simulink model "version4_dq"  (R2023b)
settings: Solver=VariableStepAuto  StartTime=0.0  StopTime=40  FixedStep=Ts_power  MaxStep=Ts_power  RelTol=1e-3
undefined symbols (not defined in the file): C_dc, c_dc, c_drt, c_f, C_hv_km, C_p_opt, Cagg, Cbase1v, H_gen, H_vsm, H_WTR, Ibase_hv, Ibase_lv, Ibase_mv, k_d_vsm, k_drt, k_p_p_vsm, k_p_q_vsm, K_pitch, ki_q, Kp_cc, kp_dc, kpu, L_comp, L_d, l_f, l_grid, L_hv_km, L_q, l_t_ehvhv, l_t_hvmv, l_t_mvlv, Lagg, lambda_opt, Lbase1v, length_export, omega_nom, omega_WTR_min, omega_WTR_n, omega_WTR_sl, phase_shift_test_state, phase_shifts, pie_export, pitch_max, pitch_min, Pitchanglevector, Powercoefficient, psi_pm, R_a, r_f, r_grid, R_hv_km, r_t_ehvhv, r_t_hvmv, r_t_mvlv, R_WTR, Ragg, rate_max, rate_min, rocof_slope ... (+22)
libraries: slpidlib x6, simulink x2, spsFirstOrderFilterLib x1, spsSampleandHoldLib x1
(part 2 of 3)

== system version4_dq/GFM+WT/CurrentControl ==
  ref : Inport
  meas : Inport  Port=2
  V grid meas : Inport  Port=3
  Constant : Constant
  Demux : Demux  Outputs=2
  Demux1 : Demux  Outputs=2
  Demux2 : Demux  Outputs=3
  Divide1 : Product  Inputs=**
  Divide2 : Product  Inputs=**
  Gain4 : Gain  Gain=l_f
  Gain5 : Gain  Gain=l_f
  Mux : Mux  Inputs=2
  Mux1 : Mux  Inputs=3
  Mux2 : Mux  Inputs=3
  PID Controller : slpidlib/PID Controller  Controller=PI  Form=Ideal  TimeDomain=Continuous-time  UseExternalTs=off  SampleTime=-1  IntegratorMethod=Forward Euler  FilterMethod=Forward Euler  ControllerParametersSource=internal  P=Kp_cc  I=1/Ti_cc  UseKiTs=off  D=0  N=100  UseFilter=on  TunerSelectOption=Transfer Function Based (PID Tuner App)  InitialConditionSource=internal  InitialConditionForIntegrator=0  InitialConditionForFilter=0  DifferentiatorICPrevScaledInput=0  ExternalReset=none  TrackingMode=off  Kt=1  LimitOutput=off  SatLimitsSource=internal  UpperSaturationLimit=inf  LowerSaturationLimit=-inf  LinearizeAsGain=on  AntiWindupMode=none  Kb=1  LimitIntegrator=off  UpperIntegratorSaturationLimit=inf  LowerIntegratorSaturationLimit=-inf  POutMin=[]  POutMax=[]  IOutMin=[]  IOutMax=[]  DOutMin=[]  DOutMax=[]  NOutMin=[]  NOutMax=[]  SumOutMin=[]  SumOutMax=[]  SaturationOutMin=[]  SaturationOutMax=[]  PParamMin=[]  PParamMax=[]  IParamMin=[]  IParamMax=[]  DParamMin=[]  DParamMax=[]  NParamMin=[]  NParamMax=[]  KbParamMin=[]  KbParamMax=[]  KtParamMin=[]  KtParamMax=[]  KbOutMin=[]  KbOutMax=[]  KtOutMin=[]  KtOutMax=[]  IntegratorOutMin=[]  IntegratorOutMax=[]  FilterOutMin=[]  FilterOutMax=[]  SumI1OutMin=[]  SumI1OutMax=[]  SumI2OutMin=[]  SumI2OutMax=[]  SumI3OutMin=[]  SumI3OutMax=[]  SumI4OutMin=[]  SumI4OutMax=[]  SumDOutMin=[]  SumDOutMax=[]  DifferentiatorOutMin=[]  DifferentiatorOutMax=[]  FilterDiffOutCoefMin=[]  FilterDiffOutCoefMax=[]  ReciprocalOutMin=[]  ReciprocalOutMax=[]  SumDenOutMin=[]  SumDenOutMax=[]  SumNumOutMin=[]  SumNumOutMax=[]  DivideOutMin=[]  DivideOutMax=[]  UdiffTsProdOutMin=[]  UdiffTsProdOutMax=[]  NTsProdOutMin=[]  NTsProdOutMax=[]  UintegralTsProdOutMin=[]  UintegralTsProdOutMax=[]  UngainTsProdOutMin=[]  UngainTsProdOutMax=[]  ClampingZeroOutDataTypeStr=Inherit: Inherit via back propagation  ClampingZeroOutMin=[]  ClampingZeroOutMax=[]  FilterDenConstantOutDataTypeStr=Inherit: Inherit via back propagation  FilterDenConstantOutMin=[]  FilterDenConstantOutMax=[]  PCopyOutDataTypeStr=Inherit: Inherit via back propagation  PCopyOutMin=[]  PCopyOutMax=[]  NCopyOutDataTypeStr=Inherit: Inherit via back propagation  NCopyOutMin=[]  NCopyOutMax=[]  IntegratorContinuousStateAttributes='Delta_v_t_q'  IntegratorStateMustResolveToSignalObject=off  IntegratorRTWStateStorageClass=Auto  FilterContinuousStateAttributes=''  FilterStateMustResolveToSignalObject=off  FilterRTWStateStorageClass=Auto  ParallelPVariant=Passthrough  IdealPVariant=InternalParameters  IVariant=InternalParameters  DVariant=Disabled  IntegratorVariant=Continuous  SatVariant=Disabled  AWVariant=Passthrough  PCopyVariant=Disabled  TRVariant=Disabled  FdbkBlocksVariant=Forward  IdealPFdbkVariant=Disabled  SatFdbkVariant=Disabled  DerivativeFilterVariant=Disabled  NVariant=Disabled  NCopyVariant=Disabled_SignalSpec  FilterICVariant=Disabled  IntegratorICVariant=InternalICs  ExternalResetVariant=Disabled  TRSumVariant=Passthrough  SumFdbkVariant=Disabled  SumVariant=Sum_PI  TsampFilterVariant=InternalTs  TsampNgainVariant=Passthrough  TsampIntegralVariant=Disabled_SignalSpec  ExternalSaturationOutDataTypeStr=Inherit: Same as second input
  PID Controller1 : slpidlib/PID Controller  Controller=PI  Form=Ideal  TimeDomain=Continuous-time  UseExternalTs=off  SampleTime=-1  IntegratorMethod=Forward Euler  FilterMethod=Forward Euler  ControllerParametersSource=internal  P=Kp_cc  I=1/Ti_cc  UseKiTs=off  D=0  N=100  UseFilter=on  TunerSelectOption=Transfer Function Based (PID Tuner App)  InitialConditionSource=internal  InitialConditionForIntegrator=1  InitialConditionForFilter=0  DifferentiatorICPrevScaledInput=0  ExternalReset=none  TrackingMode=off  Kt=1  LimitOutput=off  SatLimitsSource=internal  UpperSaturationLimit=inf  LowerSaturationLimit=-inf  LinearizeAsGain=on  AntiWindupMode=none  Kb=1  LimitIntegrator=off  UpperIntegratorSaturationLimit=inf  LowerIntegratorSaturationLimit=-inf  POutMin=[]  POutMax=[]  IOutMin=[]  IOutMax=[]  DOutMin=[]  DOutMax=[]  NOutMin=[]  NOutMax=[]  SumOutMin=[]  SumOutMax=[]  SaturationOutMin=[]  SaturationOutMax=[]  PParamMin=[]  PParamMax=[]  IParamMin=[]  IParamMax=[]  DParamMin=[]  DParamMax=[]  NParamMin=[]  NParamMax=[]  KbParamMin=[]  KbParamMax=[]  KtParamMin=[]  KtParamMax=[]  KbOutMin=[]  KbOutMax=[]  KtOutMin=[]  KtOutMax=[]  IntegratorOutMin=[]  IntegratorOutMax=[]  FilterOutMin=[]  FilterOutMax=[]  SumI1OutMin=[]  SumI1OutMax=[]  SumI2OutMin=[]  SumI2OutMax=[]  SumI3OutMin=[]  SumI3OutMax=[]  SumI4OutMin=[]  SumI4OutMax=[]  SumDOutMin=[]  SumDOutMax=[]  DifferentiatorOutMin=[]  DifferentiatorOutMax=[]  FilterDiffOutCoefMin=[]  FilterDiffOutCoefMax=[]  ReciprocalOutMin=[]  ReciprocalOutMax=[]  SumDenOutMin=[]  SumDenOutMax=[]  SumNumOutMin=[]  SumNumOutMax=[]  DivideOutMin=[]  DivideOutMax=[]  UdiffTsProdOutMin=[]  UdiffTsProdOutMax=[]  NTsProdOutMin=[]  NTsProdOutMax=[]  UintegralTsProdOutMin=[]  UintegralTsProdOutMax=[]  UngainTsProdOutMin=[]  UngainTsProdOutMax=[]  ClampingZeroOutDataTypeStr=Inherit: Inherit via back propagation  ClampingZeroOutMin=[]  ClampingZeroOutMax=[]  FilterDenConstantOutDataTypeStr=Inherit: Inherit via back propagation  FilterDenConstantOutMin=[]  FilterDenConstantOutMax=[]  PCopyOutDataTypeStr=Inherit: Inherit via back propagation  PCopyOutMin=[]  PCopyOutMax=[]  NCopyOutDataTypeStr=Inherit: Inherit via back propagation  NCopyOutMin=[]  NCopyOutMax=[]  IntegratorContinuousStateAttributes='Delta_v_t_d'  IntegratorStateMustResolveToSignalObject=off  IntegratorRTWStateStorageClass=Auto  FilterContinuousStateAttributes=''  FilterStateMustResolveToSignalObject=off  FilterRTWStateStorageClass=Auto  ParallelPVariant=Passthrough  IdealPVariant=InternalParameters  IVariant=InternalParameters  DVariant=Disabled  IntegratorVariant=Continuous  SatVariant=Disabled  AWVariant=Passthrough  PCopyVariant=Disabled  TRVariant=Disabled  FdbkBlocksVariant=Forward  IdealPFdbkVariant=Disabled  SatFdbkVariant=Disabled  DerivativeFilterVariant=Disabled  NVariant=Disabled  NCopyVariant=Disabled_SignalSpec  FilterICVariant=Disabled  IntegratorICVariant=InternalICs  ExternalResetVariant=Disabled  TRSumVariant=Passthrough  SumFdbkVariant=Disabled  SumVariant=Sum_PI  TsampFilterVariant=InternalTs  TsampNgainVariant=Passthrough  TsampIntegralVariant=Disabled_SignalSpec  ExternalSaturationOutDataTypeStr=Inherit: Same as second input
  Step1 : Step  Before=1  SampleTime=0
  Step2 : Step  Before=1  SampleTime=0
  Sum1 : Sum  Inputs=|+-
  Sum2 : Sum  Inputs=+-|
  Sum4 : Sum  Inputs=++-
  Sum5 : Sum  Inputs=+++
  Transfer Fcn2 : TransferFcn  Commented=on  Denominator=[0.005 1]
  Transfer Fcn3 : TransferFcn  Commented=on  Denominator=[0.005 1]
  d-axis-control : Scope  Commented=on  NumInputPorts=3
  q-axis control : Scope  Commented=on  NumInputPorts=3
  v_m : Outport
  wires:
  Mux/1 -> v_m/1
  Sum1/1 -> Divide2/1, d-axis-control/1
  ref/1 -> Demux/1
  meas/1 -> Demux1/1
  Demux1/2 -> Gain5/1, Sum2/2
  Demux1/1 -> Gain4/1, Sum1/2
  Demux/2 -> Sum2/1
  Demux/1 -> Sum1/1
  PID Controller/1 -> Mux2/2, Sum5/2
  Sum4/1 -> d-axis-control/3, Mux/1
  Gain5/1 -> Mux1/3, Sum4/3
  Gain4/1 -> Mux2/3, Sum5/1
  Demux2/2 -> Transfer Fcn3/1
  Sum5/1 -> q-axis control/3, Mux/2
  V grid meas/1 -> Demux2/1
  Demux2/1 -> Transfer Fcn2/1
  Transfer Fcn2/1 -> Mux1/1, Sum4/1
  Mux1/1 -> d-axis-control/2
  Mux2/1 -> q-axis control/2
  Transfer Fcn3/1 -> Mux2/1, Sum5/3
  PID Controller1/1 -> Sum4/2, Mux1/2
  Sum2/1 -> q-axis control/1, Divide1/1
  Step2/1 -> Divide1/2
  Divide1/1 -> PID Controller/1
  Step1/1 -> Divide2/2
  Divide2/1 -> PID Controller1/1

== system version4_dq/GFM+WT/DC-link voltage controller ==
  ref : Inport
  meas : Inport  Port=2
  Mux : Mux  Inputs=2
  PID Controller : slpidlib/PID Controller  Controller=PI  Form=Ideal  TimeDomain=Continuous-time  UseExternalTs=off  SampleTime=-1  IntegratorMethod=Forward Euler  FilterMethod=Forward Euler  ControllerParametersSource=internal  P=kp_dc  I=1/Ti_dc  UseKiTs=off  D=0.0506  N=100  UseFilter=on  TunerSelectOption=Transfer Function Based (PID Tuner App)  InitialConditionSource=internal  InitialConditionForIntegrator=0  InitialConditionForFilter=0  DifferentiatorICPrevScaledInput=0  ExternalReset=none  TrackingMode=off  Kt=1  LimitOutput=off  SatLimitsSource=internal  UpperSaturationLimit=0.5  LowerSaturationLimit=-0.5  LinearizeAsGain=on  AntiWindupMode=clamping  Kb=1  LimitIntegrator=off  UpperIntegratorSaturationLimit=0.5  LowerIntegratorSaturationLimit=-0.5  POutMin=[]  POutMax=[]  IOutMin=[]  IOutMax=[]  DOutMin=[]  DOutMax=[]  NOutMin=[]  NOutMax=[]  SumOutMin=[]  SumOutMax=[]  SaturationOutMin=[]  SaturationOutMax=[]  PParamMin=[]  PParamMax=[]  IParamMin=[]  IParamMax=[]  DParamMin=[]  DParamMax=[]  NParamMin=[]  NParamMax=[]  KbParamMin=[]  KbParamMax=[]  KtParamMin=[]  KtParamMax=[]  KbOutMin=[]  KbOutMax=[]  KtOutMin=[]  KtOutMax=[]  IntegratorOutMin=[]  IntegratorOutMax=[]  FilterOutMin=[]  FilterOutMax=[]  SumI1OutMin=[]  SumI1OutMax=[]  SumI2OutMin=[]  SumI2OutMax=[]  SumI3OutMin=[]  SumI3OutMax=[]  SumI4OutMin=[]  SumI4OutMax=[]  SumDOutMin=[]  SumDOutMax=[]  DifferentiatorOutMin=[]  DifferentiatorOutMax=[]  FilterDiffOutCoefMin=[]  FilterDiffOutCoefMax=[]  ReciprocalOutMin=[]  ReciprocalOutMax=[]  SumDenOutMin=[]  SumDenOutMax=[]  SumNumOutMin=[]  SumNumOutMax=[]  DivideOutMin=[]  DivideOutMax=[]  UdiffTsProdOutMin=[]  UdiffTsProdOutMax=[]  NTsProdOutMin=[]  NTsProdOutMax=[]  UintegralTsProdOutMin=[]  UintegralTsProdOutMax=[]  UngainTsProdOutMin=[]  UngainTsProdOutMax=[]  ClampingZeroOutDataTypeStr=Inherit: Inherit via back propagation  ClampingZeroOutMin=[]  ClampingZeroOutMax=[]  FilterDenConstantOutDataTypeStr=Inherit: Inherit via back propagation  FilterDenConstantOutMin=[]  FilterDenConstantOutMax=[]  PCopyOutDataTypeStr=Inherit: Inherit via back propagation  PCopyOutMin=[]  PCopyOutMax=[]  NCopyOutDataTypeStr=Inherit: Inherit via back propagation  NCopyOutMin=[]  NCopyOutMax=[]  IntegratorContinuousStateAttributes='Delta_P_msc'  IntegratorStateMustResolveToSignalObject=off  IntegratorRTWStateStorageClass=Auto  FilterContinuousStateAttributes=''  FilterStateMustResolveToSignalObject=off  FilterRTWStateStorageClass=Auto  ParallelPVariant=Passthrough  IdealPVariant=InternalParameters  IVariant=InternalParameters  DVariant=Disabled  IntegratorVariant=Continuous  SatVariant=Disabled  AWVariant=Passthrough  PCopyVariant=Disabled  TRVariant=Disabled  FdbkBlocksVariant=Forward  IdealPFdbkVariant=Disabled  SatFdbkVariant=Disabled  DerivativeFilterVariant=Disabled  NVariant=Disabled  NCopyVariant=Disabled_SignalSpec  FilterICVariant=Disabled  IntegratorICVariant=InternalICs  ExternalResetVariant=Disabled  TRSumVariant=Passthrough  SumFdbkVariant=Disabled  SumVariant=Sum_PI  TsampFilterVariant=InternalTs  TsampNgainVariant=Passthrough  TsampIntegralVariant=Disabled_SignalSpec  ExternalSaturationOutDataTypeStr=Inherit: Same as second input
  Square : Math  Operator=square
  Square1 : Math  Operator=square
  Sum : Sum  Inputs=+-|
  input : Outport
  error : Outport  Port=2
  out : Outport  Port=3
  Out4 : Outport  Port=4
  wires:
  Mux/1 -> input/1
  PID Controller/1 -> Out4/1, out/1
  meas/1 -> Square/1
  ref/1 -> Square1/1
  Square/1 -> Mux/2, Sum/2
  Square1/1 -> Mux/1, Sum/1
  Sum/1 -> PID Controller/1, error/1

== system version4_dq/GFM+WT/PLL>>grid1 ==
  note: inv ([  cos(wt)   sin(wt)
      |    -sin(wt)    cos(wt)   ])
  note: =
  note: [  al
      |     be  ]
  note: =
  note: [  al
      |     be  ]
  note: [ d
      |    q ]
  note: *
  note: [ d
      |    q ]
  note: [  cos(wt)   -sin(wt)
      |    sin(wt)    cos(wt)   ]
  note: *
  v_t_dq : Inport
  thetaPLL : Inport  Port=2
  Cos : Trigonometry  Operator=cos
  Demux1 : Demux  Outputs=2
  Display5 : Display
  Mux3 : Mux  Inputs=2
  Product{,1..3} (4 alike) : Product
  Sin : Trigonometry
  Sum : Sum  Inputs=+-
  Sum1 : Sum
  v_t_DQ : Outport  InitialOutput=[0,0]  VectorParamsAs1DForOutWhenUnconnected=off
  wires:
  v_t_dq/1 -> Demux1/1
  thetaPLL/1 -> Cos/1, Sin/1
  Sin/1 -> Product3/2, Product1/2
  Demux1/1 -> Product3/1, Product/1
  Cos/1 -> Product2/2, Product/2
  Product/1 -> Sum/1
  Demux1/2 -> Product2/1, Product1/1
  Product1/1 -> Sum/2
  Sum/1 -> Mux3/1
  Product2/1 -> Sum1/1
  Product3/1 -> Sum1/2
  Sum1/1 -> Mux3/2
  Mux3/1 -> Display5/1, v_t_DQ/1

== system version4_dq/GFM+WT/PQ PCC ==
  note: PQ VSC bus
  IDQ : Inport
  VDQ : Inport  Port=2
  Demux7 : Demux  Outputs=[vect vect]
  Demux8 : Demux  Outputs=[vect vect]
  Product{1,3..5} (4 alike) : Product  InputSameDT=on  SaturateOnIntegerOverflow=on  OutDataTypeStr=Inherit: Same as first input
  Sum : Sum  InputSameDT=on  SaturateOnIntegerOverflow=on  OutDataTypeStr=Inherit: Same as first input
  Sum1 : Sum  Inputs=+-  InputSameDT=on  SaturateOnIntegerOverflow=on  OutDataTypeStr=Inherit: Same as first input
  P : Outport
  Q : Outport  Port=2
  wires:
  Product5/1 -> Sum1/2
  Product1/1 -> Sum1/1
  Demux8/2 -> Product1/1, Product4/1
  Demux7/1 -> Product1/2, Product3/1
  Demux8/1 -> Product5/1, Product3/2
  Product4/1 -> Sum/2
  Demux7/2 -> Product4/2, Product5/2
  Product3/1 -> Sum/1
  VDQ/1 -> Demux8/1
  Sum1/1 -> Q/1
  IDQ/1 -> Demux7/1
  Sum/1 -> P/1

== system version4_dq/GFM+WT/RL filter1 ==
  note: Inverter side inductor
  v_vsc_D : Inport
  v_t_D : Inport  Port=2
  v_t_Q : Inport  Port=3
  v_vsc_Q : Inport  Port=4
  In5 : Inport  Port=5
  1 : Gain  Gain=r_f*Zbase1v
  2 : Gain  Gain=1/(l_f*Lbase1v)
  3 : Gain  Gain=r_f*Zbase1v
  4 : Gain  Gain=1/(l_f*Lbase1v)
  Id : Scope
  Id_int : Integrator  UpperSaturationLimit=50  LowerSaturationLimit=-1000
  Iq : Scope
  Iq_int : Integrator  UpperSaturationLimit=50  LowerSaturationLimit=-1000
  L value : Constant  Value=l_f*Lbase1v  SampleTime=-1
  Product : Product
  Product1 : Product
  Product2 : Product
  Sum1 : Sum  Inputs=|+---
  Sum8 : Sum  Inputs=|+-+-
  id1 : Display
  iD : Outport
  iQ : Outport  Port=2
  wires:
  In5/1 -> Product/1
  Product/1 -> [wL], id1/1
  L value/1 -> Product/2
  v_vsc_Q/1 -> Sum1/2
  v_t_Q/1 -> Sum1/1
  v_vsc_D/1 -> Sum8/2
  v_t_D/1 -> Sum8/1
  Product2/1 -> Sum8/3
  Iq_int/1 -> iQ/1, 3/1, Iq/1, Product2/2
  4/1 -> Iq_int/1
  Sum8/1 -> 2/1
  2/1 -> Id_int/1
  Sum1/1 -> 4/1
  3/1 -> Sum1/4
  Product1/1 -> Sum1/3
  1/1 -> Sum8/4
  Id_int/1 -> iD/1, Product1/2, Id/1, 1/1
  [wL] -> Product1/1, Product2/1

== system version4_dq/GFM+WT/SwingEqVer1 ==
  Pref : Inport
  Pm : Inport  Port=2
  Constant6 : Constant  Value=omega_nom
  Gain1 : Gain  Gain=1/(2*pi)
  Gain2 : Gain  Gain=180/pi
  Gain3 : Gain  Gain=1/(2*H_vsm)
  Gain4 : Gain  Gain=omega_nom
  Gain6 : Gain  Commented=through  Gain=k_p_p_vsm
  Gain7 : Gain  Gain=180/pi
  Gain8 : Gain  Gain=k_d_vsm
  Integrator : Integrator  WrappedStateUpperValue=2*pi  WrappedStateLowerValue=0  ContinuousStateAttributes='Delta_theta_vsm'
  Integrator1 : Integrator  WrappedStateUpperValue=2*pi  WrappedStateLowerValue=0
  Integrator2 : Integrator  ContinuousStateAttributes='Delta_omega_vsm'
  Sum1 : Sum  Inputs=+-|
  Sum2 : Sum  Inputs=++|
  Sum3 : Sum  Inputs=-+|
  Sum7 : Sum  Inputs=|+-
  To Workspace : ToWorkspace  Commented=on  VariableName=GFM_freq  SaveFormat=Structure With Time  SampleTime=-1
  Transfer Fcn : TransferFcn  Denominator=[2*H_vsm k_d_vsm]
  vsm : Scope  NumInputPorts=3
  theta_vsm_rad : Outport
  Omega_ref : Outport  Port=2
  wires:
  Sum1/1 -> Sum7/1, vsm/1  "delta P"
  Sum2/1 -> Gain1/1, Omega_ref/1, Integrator/1  "omega_ref"
  Integrator2/1 -> Gain6/1, Gain8/1
  Gain6/1 -> Gain4/1  "Delta_omega"
  Pm/1 -> Sum1/2
  Gain7/1 -> Sum3/2  "theta_ref_deg"
  Pref/1 -> Sum1/1
  Constant6/1 -> Integrator1/1
  Gain4/1 -> Sum2/2
  Gain1/1 -> vsm/2, To Workspace/1  "Frequency"
  Integrator1/1 -> Gain2/1  "theta_ref_rad"
  Gain2/1 -> Sum3/1  "theta_ref_deg"
  Integrator/1 -> theta_vsm_rad/1, Gain7/1
  Gain8/1 -> Sum7/2
  Gain3/1 -> Integrator2/1
  Sum7/1 -> Gain3/1  "delta P"
  Sum3/1 -> vsm/3  "omega_ref"

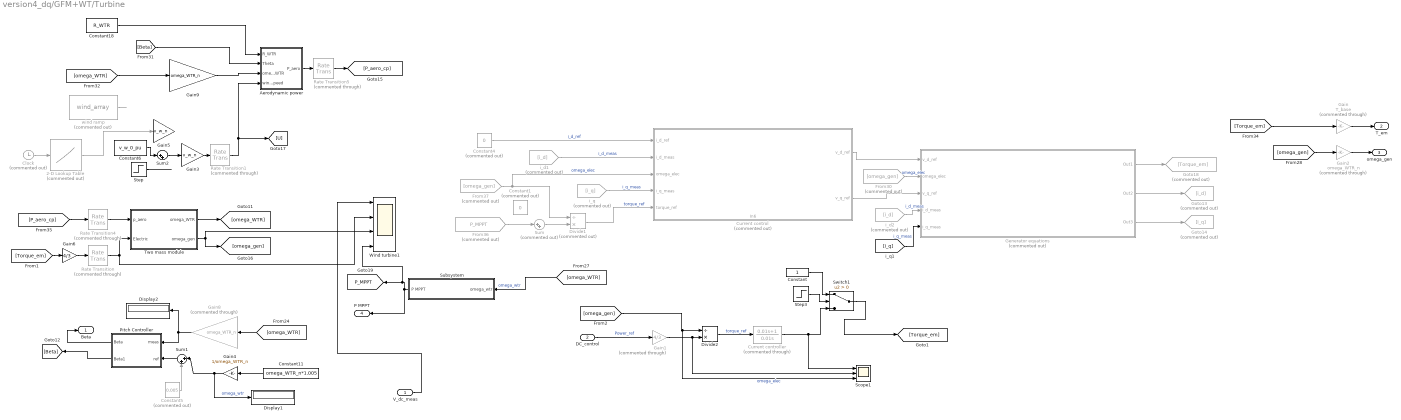
== system version4_dq/GFM+WT/Turbine ==
  V_dc_meas : Inport
  DC_control : Inport  Port=2
  2-D Lookup Table : Lookup_n-D  Commented=on  NumberOfTableDimensions=1  BreakpointsForDimension1=wind_array_step(1,:)  BreakpointsForDimension2=[1:3]  IndexSearchMethod=Linear search  Table=wind_array_step(2,:)  InterpMethod=Nearest  InternalRulePriority=Speed  RndMeth=Simplest
  Aerodynamic power : Subsystem
  Clock : Clock  Commented=on
  Constant : Constant
  Constant1 : Constant  Commented=on  Value=0
  Constant11 : Constant  Value=omega_WTR_n*1.005
  Constant18 : Constant  Value=R_WTR
  Constant4 : Constant  Commented=on  Value=0
  Constant5 : Constant  Commented=on  Value=0.005
  Constant6 : Constant  Value=v_w_0_pu
  Current control : Subsystem  Commented=on
      settings: PortSchema="{\"entries\":[{\"content\":{\"sides\":[{\"content\":{\"connectorIds\":[\"In1\",\"In2\",\"In3\",\"In4\",\"In5\"]},\"type\":\"ConnectorPlacement.EquallySpacedRectSide\",\"uuid\":\"f0c0ebaa-c967-4356-ac1b-c57f63a29779\"},{\"content\":{\"connectorIds\":[\"Out1\",\"Out2\"],\"side\":\"RIGHT\"},\"type\":\"ConnectorPlacement.EquallySpacedRectSide\",\"uuid\":\"1cdf54d9-8841-4054-96d8-98f023823611\"},{\"content\":{\"side\":\"TOP\"},\"type\":\"ConnectorPlacement.EquallySpacedRectSide\",\"uuid\":\"e5446ced-f102-4515-b1a2-d62d39d31328\"},{\"content\":{\"connectorIds\":[\"In6\"],\"side\":\"BOTTOM\"},\"type\":\"ConnectorPlacement.EquallySpacedRectSide\",\"uuid\":\"501a05db-372f-49fd-99c3-d79253c332da\"}]},\"type\":\"ConnectorPlacement.EquallySpacedConnector\",\"uuid\":\"99b5cc9b-ee78-4a5c-8cde-7a0c5c1e273f\"}],\"packageUris\":[\"http://schema.mathworks.com/mf0/Connector/R2020b\"],\"version\":\"1.0\"}"
  Current controller : TransferFcn  Commented=through  Numerator=[0.01 1]  Denominator=[0.01 0]
  Display1 : Display
  Display2 : Display
  Divide1 : Product  Commented=on  Inputs=/*
  Divide2 : Product  Inputs=/*
  From30 : From  Commented=on  GotoTag=omega_gen
  From36 : From  Commented=on  GotoTag=P_MPPT
  From37 : From  Commented=on  GotoTag=omega_gen
  Gain : Gain  Commented=through  Gain=T_base
  Gain1 : Gain  Commented=through  Gain=4/3
  Gain2 : Gain  Commented=through  Gain=omega_WTR_n
  Gain3 : Gain  Gain=v_w_n
  Gain4 : Gain  Gain=1/omega_WTR_n
  Gain5 : Gain  Gain=v_w_n
  Gain6 : Gain  Gain=4/3
  Gain8 : Gain  Commented=through  Gain=omega_WTR_n
  Gain9 : Gain  Gain=omega_WTR_n
  Generator equations : Subsystem  Commented=on
  Goto13 : Goto  Commented=on  GotoTag=i_d
  Goto14 : Goto  Commented=on  GotoTag=i_q
  Goto18 : Goto  Commented=on  GotoTag=Torque_em
  Pitch Controller : Subsystem
  Rate Transition : RateTransition  Commented=through  OutPortSampleTime=100e-6
  Rate Transition1 : RateTransition  Commented=through  OutPortSampleTime=50e-6
  Rate Transition4 : RateTransition  Commented=through  OutPortSampleTime=100e-6
  Rate Transition5 : RateTransition  Commented=through  OutPortSampleTime=100e-6
  Scope1 : Scope  NumInputPorts=3
  Step : Step  Time=15  Before=1.34  After=1.34  SampleTime=0
  Step3 : Step  Time=3  After=0  SampleTime=0
  Subsystem : Subsystem
  Sum : Sum  Commented=on  Inputs=|++
  Sum1 : Sum  Inputs=|++
  Sum2 : Sum  Inputs=|++
  Switch1 : Switch  Criteria=u2 > Threshold  SaturateOnIntegerOverflow=off  InputSameDT=off
  Two mass module : Subsystem
  Wind turbine1 : Scope  NumInputPorts=4
  i_d1 : From  Commented=on  GotoTag=i_d
  i_d2 : From  Commented=on  GotoTag=i_d
  i_q : From  Commented=on  GotoTag=i_q
  wind ramp : FromWorkspace  Commented=on  VariableName=wind_array
  Beta : Outport
  T_em : Outport  Port=2
  omega_gen : Outport  Port=3
  P MPPT : Outport  Port=4
  tag scope: P_MPPT=global
  wires:
  [omega_gen] -> Gain2/1
  [omega_WTR] -> Subsystem/1(omega_wtr)  "omega_wtr"
  i_d1/1 -> Current control/2(i_d_meas)  "i_d_meas"
  Generator equations/3(Out3) -> Goto14/1
  [i_q] -> Generator equations/5(i_q_meas)  "i_q_meas"
  Pitch Controller/1(Beta) -> Beta/1
  i_d2/1 -> Generator equations/4(i_d_meas)  "i_d_meas"
  Constant18/1 -> Aerodynamic power/1(R_WTR)
  From30/1 -> Generator equations/2(omega_elec)  "omega_elec"
  Rate Transition1/1 -> Aerodynamic power/4(wind speed), [U]
  [Torque_em] -> Gain6/1
  Constant11/1 -> Gain4/1
  wind ramp/1 -> ?
  [P_aero_cp] -> Rate Transition4/1
  Constant4/1 -> Current control/1(i_d_ref)  "i_d_ref"
  Generator equations/1(Out1) -> Goto18/1
  Constant5/1 -> Sum1/2
  Two mass module/1(omega_WTR) -> [omega_WTR]
  From36/1 -> Sum/1
  Two mass module/2(omega_gen) -> Wind turbine1/3, [omega_gen]
  From37/1 -> Divide1/1, Current control/3(omega_elec)  "omega_elec"
  Sum1/1 -> Pitch Controller/2(ref)
  Gain4/1 -> Sum1/1, Display1/1  "omega_wtr"
  Constant6/1 -> Sum2/1
  [omega_WTR] -> Gain8/1
  Clock/1 -> 2-D Lookup Table/1
  Pitch Controller/2(Beta1) -> [Beta]
  i_q/1 -> Current control/4(i_q_meas)  "i_q_meas"
  Aerodynamic power/1(P_aero) -> Rate Transition5/1
  Gain9/1 -> Aerodynamic power/3(omega_WTR)
  Gain8/1 -> Display2/1, Pitch Controller/1(meas)
  [Beta] -> Aerodynamic power/2(Theta)
  2-D Lookup Table/1 -> Gain5/1
  Subsystem/1(P MPPT) -> P MPPT/1, Wind turbine1/4, [P_MPPT]
  Divide1/1 -> Current control/5(torque_ref)  "torque_ref"
  Current control/1(v_d_ref) -> Generator equations/1(v_d_ref)
  Generator equations/2(Out2) -> Goto13/1
  [omega_WTR] -> Gain9/1
  Current control/2(v_q_ref) -> Generator equations/3(v_q_ref)
  Gain/1 -> T_em/1
  Gain2/1 -> omega_gen/1
  Sum/1 -> Divide1/2
  ? -> ?
  [omega_gen] -> Scope1/3, Divide2/1  "omega_elec"
  V_dc_meas/1 -> Wind turbine1/1
  Current controller/1 -> Switch1/3, Scope1/1
  Divide2/1 -> Current controller/1  "torque_ref"
  DC_control/1 -> Gain1/1  "Power_ref"
  Step3/1 -> Switch1/2
  Constant/1 -> Switch1/1
  Rate Transition/1 -> Wind turbine1/2, Two mass module/2(Electric)
  Gain3/1 -> Rate Transition1/1
  Rate Transition4/1 -> Two mass module/1(p_aero)
  Rate Transition5/1 -> [P_aero_cp]
  Gain1/1 -> Scope1/2, Divide2/2
  Switch1/1 -> [Torque_em]
  [Torque_em] -> Gain/1
  Gain6/1 -> Rate Transition/1
  Sum2/1 -> Gain3/1
  Step/1 -> ?

== system version4_dq/GFM+WT/Voltage control ==
  Qm : Inport
  Qref : Inport  Port=2
  Constant5 : Constant
  Gain9 : Gain  Gain=k_p_q_vsm
  Qdroop : Scope  NumInputPorts=2
  Scope : Scope  NumInputPorts=4
  Sum3 : Sum  Inputs=|-+
  Sum4 : Sum  Inputs=|++
  Transfer Fcn1 : TransferFcn  Numerator=[ki_q]  Denominator=[1 ki_q]  ContinuousStateAttributes='Delta_Q'
  Vref : Outport
  delta Q : Outport  Port=2
  wires:
  Constant5/1 -> Sum4/2
  Gain9/1 -> Scope/3, Sum4/1
  Transfer Fcn1/1 -> Scope/2, Gain9/1
  Sum3/1 -> Transfer Fcn1/1, Scope/1, Qdroop/2, delta Q/1  "delta Q"
  Sum4/1 -> Scope/4, Qdroop/1, Vref/1  "Vref"
  Qref/1 -> Sum3/2
  Qm/1 -> Sum3/1

== system version4_dq/GFM+WT/VoltageControl ==
  ref : Inport
  meas : Inport  Port=2
  I filter meas : Inport  Port=3
  Constant : Constant  Value=0
  Demux1 : Demux  Outputs=2
  Demux2 : Demux  Outputs=3
  Demux3 : Demux  Outputs=2
  Gain4 : Gain  Gain=c_f
  Gain5 : Gain  Gain=c_f
  Mux : Mux  Inputs=2
  Mux1 : Mux  Inputs=3
  Mux2 : Mux  Inputs=3
  PID Controller : slpidlib/PID Controller  Controller=PI  Form=Ideal  TimeDomain=Continuous-time  UseExternalTs=off  SampleTime=-1  IntegratorMethod=Forward Euler  FilterMethod=Forward Euler  ControllerParametersSource=internal  P=kpu  I=1/Tnu  UseKiTs=off  D=0  N=100  UseFilter=on  TunerSelectOption=Transfer Function Based (PID Tuner App)  InitialConditionSource=internal  InitialConditionForIntegrator=0  InitialConditionForFilter=0  DifferentiatorICPrevScaledInput=0  ExternalReset=none  TrackingMode=off  Kt=1  LimitOutput=off  SatLimitsSource=internal  UpperSaturationLimit=2  LowerSaturationLimit=-2  LinearizeAsGain=off  AntiWindupMode=none  Kb=1  LimitIntegrator=off  UpperIntegratorSaturationLimit=inf  LowerIntegratorSaturationLimit=-inf  POutMin=[]  POutMax=[]  IOutMin=[]  IOutMax=[]  DOutMin=[]  DOutMax=[]  NOutMin=[]  NOutMax=[]  SumOutMin=[]  SumOutMax=[]  SaturationOutMin=[]  SaturationOutMax=[]  PParamMin=[]  PParamMax=[]  IParamMin=[]  IParamMax=[]  DParamMin=[]  DParamMax=[]  NParamMin=[]  NParamMax=[]  KbParamMin=[]  KbParamMax=[]  KtParamMin=[]  KtParamMax=[]  KbOutMin=[]  KbOutMax=[]  KtOutMin=[]  KtOutMax=[]  IntegratorOutMin=[]  IntegratorOutMax=[]  FilterOutMin=[]  FilterOutMax=[]  SumI1OutMin=[]  SumI1OutMax=[]  SumI2OutMin=[]  SumI2OutMax=[]  SumI3OutMin=[]  SumI3OutMax=[]  SumI4OutMin=[]  SumI4OutMax=[]  SumDOutMin=[]  SumDOutMax=[]  DifferentiatorOutMin=[]  DifferentiatorOutMax=[]  FilterDiffOutCoefMin=[]  FilterDiffOutCoefMax=[]  ReciprocalOutMin=[]  ReciprocalOutMax=[]  SumDenOutMin=[]  SumDenOutMax=[]  SumNumOutMin=[]  SumNumOutMax=[]  DivideOutMin=[]  DivideOutMax=[]  UdiffTsProdOutMin=[]  UdiffTsProdOutMax=[]  NTsProdOutMin=[]  NTsProdOutMax=[]  UintegralTsProdOutMin=[]  UintegralTsProdOutMax=[]  UngainTsProdOutMin=[]  UngainTsProdOutMax=[]  ClampingZeroOutDataTypeStr=Inherit: Inherit via back propagation  ClampingZeroOutMin=[]  ClampingZeroOutMax=[]  FilterDenConstantOutDataTypeStr=Inherit: Inherit via back propagation  FilterDenConstantOutMin=[]  FilterDenConstantOutMax=[]  PCopyOutDataTypeStr=Inherit: Inherit via back propagation  PCopyOutMin=[]  PCopyOutMax=[]  NCopyOutDataTypeStr=Inherit: Inherit via back propagation  NCopyOutMin=[]  NCopyOutMax=[]  IntegratorContinuousStateAttributes='Delta_i_ref_q'  IntegratorStateMustResolveToSignalObject=off  IntegratorRTWStateStorageClass=Auto  FilterContinuousStateAttributes=''  FilterStateMustResolveToSignalObject=off  FilterRTWStateStorageClass=Auto  ParallelPVariant=Passthrough  IdealPVariant=InternalParameters  IVariant=InternalParameters  DVariant=Disabled  IntegratorVariant=Continuous  SatVariant=Disabled  AWVariant=Passthrough  PCopyVariant=Disabled  TRVariant=Disabled  FdbkBlocksVariant=Forward  IdealPFdbkVariant=Disabled  SatFdbkVariant=Disabled  DerivativeFilterVariant=Disabled  NVariant=Disabled  NCopyVariant=Disabled_SignalSpec  FilterICVariant=Disabled  IntegratorICVariant=InternalICs  ExternalResetVariant=Disabled  TRSumVariant=Passthrough  SumFdbkVariant=Disabled  SumVariant=Sum_PI  TsampFilterVariant=InternalTs  TsampNgainVariant=Passthrough  TsampIntegralVariant=Disabled_SignalSpec  ExternalSaturationOutDataTypeStr=Inherit: Same as second input
  PID Controller1 : slpidlib/PID Controller  Controller=PI  Form=Ideal  TimeDomain=Continuous-time  UseExternalTs=off  SampleTime=-1  IntegratorMethod=Forward Euler  FilterMethod=Forward Euler  ControllerParametersSource=internal  P=kpu  I=1/Tnu  UseKiTs=off  D=0  N=100  UseFilter=on  TunerSelectOption=Transfer Function Based (PID Tuner App)  InitialConditionSource=internal  InitialConditionForIntegrator=1  InitialConditionForFilter=0  DifferentiatorICPrevScaledInput=0  ExternalReset=none  TrackingMode=off  Kt=1  LimitOutput=off  SatLimitsSource=internal  UpperSaturationLimit=2  LowerSaturationLimit=-2  LinearizeAsGain=off  AntiWindupMode=none  Kb=1  LimitIntegrator=off  UpperIntegratorSaturationLimit=inf  LowerIntegratorSaturationLimit=-inf  POutMin=[]  POutMax=[]  IOutMin=[]  IOutMax=[]  DOutMin=[]  DOutMax=[]  NOutMin=[]  NOutMax=[]  SumOutMin=[]  SumOutMax=[]  SaturationOutMin=[]  SaturationOutMax=[]  PParamMin=[]  PParamMax=[]  IParamMin=[]  IParamMax=[]  DParamMin=[]  DParamMax=[]  NParamMin=[]  NParamMax=[]  KbParamMin=[]  KbParamMax=[]  KtParamMin=[]  KtParamMax=[]  KbOutMin=[]  KbOutMax=[]  KtOutMin=[]  KtOutMax=[]  IntegratorOutMin=[]  IntegratorOutMax=[]  FilterOutMin=[]  FilterOutMax=[]  SumI1OutMin=[]  SumI1OutMax=[]  SumI2OutMin=[]  SumI2OutMax=[]  SumI3OutMin=[]  SumI3OutMax=[]  SumI4OutMin=[]  SumI4OutMax=[]  SumDOutMin=[]  SumDOutMax=[]  DifferentiatorOutMin=[]  DifferentiatorOutMax=[]  FilterDiffOutCoefMin=[]  FilterDiffOutCoefMax=[]  ReciprocalOutMin=[]  ReciprocalOutMax=[]  SumDenOutMin=[]  SumDenOutMax=[]  SumNumOutMin=[]  SumNumOutMax=[]  DivideOutMin=[]  DivideOutMax=[]  UdiffTsProdOutMin=[]  UdiffTsProdOutMax=[]  NTsProdOutMin=[]  NTsProdOutMax=[]  UintegralTsProdOutMin=[]  UintegralTsProdOutMax=[]  UngainTsProdOutMin=[]  UngainTsProdOutMax=[]  ClampingZeroOutDataTypeStr=Inherit: Inherit via back propagation  ClampingZeroOutMin=[]  ClampingZeroOutMax=[]  FilterDenConstantOutDataTypeStr=Inherit: Inherit via back propagation  FilterDenConstantOutMin=[]  FilterDenConstantOutMax=[]  PCopyOutDataTypeStr=Inherit: Inherit via back propagation  PCopyOutMin=[]  PCopyOutMax=[]  NCopyOutDataTypeStr=Inherit: Inherit via back propagation  NCopyOutMin=[]  NCopyOutMax=[]  IntegratorContinuousStateAttributes='Delta_i_ref_d'  IntegratorStateMustResolveToSignalObject=off  IntegratorRTWStateStorageClass=Auto  FilterContinuousStateAttributes=''  FilterStateMustResolveToSignalObject=off  FilterRTWStateStorageClass=Auto  ParallelPVariant=Passthrough  IdealPVariant=InternalParameters  IVariant=InternalParameters  DVariant=Disabled  IntegratorVariant=Continuous  SatVariant=Disabled  AWVariant=Passthrough  PCopyVariant=Disabled  TRVariant=Disabled  FdbkBlocksVariant=Forward  IdealPFdbkVariant=Disabled  SatFdbkVariant=Disabled  DerivativeFilterVariant=Disabled  NVariant=Disabled  NCopyVariant=Disabled_SignalSpec  FilterICVariant=Disabled  IntegratorICVariant=InternalICs  ExternalResetVariant=Disabled  TRSumVariant=Passthrough  SumFdbkVariant=Disabled  SumVariant=Sum_PI  TsampFilterVariant=InternalTs  TsampNgainVariant=Passthrough  TsampIntegralVariant=Disabled_SignalSpec  ExternalSaturationOutDataTypeStr=Inherit: Same as second input
  Sum1 : Sum  Inputs=|+-
  Sum2 : Sum  Inputs=+-|
  Sum4 : Sum  Inputs=++-
  Sum5 : Sum  Inputs=+++
  Transfer Fcn2 : TransferFcn  Commented=on  Denominator=[0.005 1]
  Transfer Fcn3 : TransferFcn  Commented=on  Denominator=[0.005 1]
  d-axis v control : Scope  NumInputPorts=3
  q-axis v control : Scope  NumInputPorts=3
  Out1 : Outport
  wires:
  Demux2/1 -> Transfer Fcn3/1
  I filter meas/1 -> Demux2/1
  Sum5/1 -> Mux/2, q-axis v control/3
  Demux2/2 -> Transfer Fcn2/1
  Sum4/1 -> Mux/1, d-axis v control/3
  Sum2/1 -> PID Controller/1, q-axis v control/1
  PID Controller/1 -> Mux1/2, Sum5/2
  Demux3/1 -> Sum1/1
  Demux3/2 -> Sum2/1
  Demux1/2 -> Gain4/1, Sum2/2
  meas/1 -> Demux1/1
  Sum1/1 -> PID Controller1/1, d-axis v control/1
  Mux/1 -> Out1/1
  Demux2/3 -> ?
  Gain4/1 -> Mux2/3, Sum4/3
  Gain5/1 -> Mux1/3, Sum5/1
  Demux1/1 -> Sum1/2, Gain5/1
  PID Controller1/1 -> Mux2/2, Sum4/2
  Transfer Fcn3/1 -> Mux2/1, Sum4/1
  Mux1/1 -> q-axis v control/2
  Mux2/1 -> d-axis v control/2
  Transfer Fcn2/1 -> Sum5/3, Mux1/1
  ref/1 -> Demux3/1

== system version4_dq/GFM+WT/grid>>PLL1 ==
  note: [  al
      |     be  ]
  note: [ d
      |    q ]
  note: [  cos(wt)   -sin(wt)
      |    sin(wt)    cos(wt)   ]
  note: =
  note: *
  note: [  al
      |     be  ]
  note: [ d
      |    q ]
  note: inv ([  cos(wt)   sin(wt)
      |    -sin(wt)    cos(wt)   ])
  note: =
  note: *
  i_vsc_DQ : Inport
  wt : Inport  Port=2
  Cos : Trigonometry  Operator=cos
  Demux1 : Demux  Outputs=[vect vect]
  Display5 : Display
  Mux3 : Mux  Inputs=2
  Product{,1..3} (4 alike) : Product
  Sin : Trigonometry
  Sum : Sum
  Sum1 : Sum  Inputs=+-
  vgdq : Outport  InitialOutput=[0,0]  VectorParamsAs1DForOutWhenUnconnected=off
  wires:
  Product3/1 -> Sum1/2
  Demux1/2 -> Product2/1, Product1/1
  Product2/1 -> Sum1/1
  Cos/1 -> Product2/2, Product/2
  Product1/1 -> Sum/2
  Sin/1 -> Product3/2, Product1/2
  i_vsc_DQ/1 -> Demux1/1
  Sum1/1 -> Mux3/2
  Mux3/1 -> vgdq/1, Display5/1
  Sum/1 -> Mux3/1
  Product/1 -> Sum/1
  wt/1 -> Cos/1, Sin/1
  Demux1/1 -> Product3/1, Product/1

== system version4_dq/GFM+WT/grid>>PLL2 ==
  note: *
  note: =
  note: inv ([  cos(wt)   sin(wt)
      |    -sin(wt)    cos(wt)   ])
  note: [ d
      |    q ]
  note: [  al
      |     be  ]
  note: *
  note: =
  note: [  cos(wt)   -sin(wt)
      |    sin(wt)    cos(wt)   ]
  note: [ d
      |    q ]
  note: [  al
      |     be  ]
  v_vsc_DQ : Inport
  wt : Inport  Port=2
  Cos : Trigonometry  Operator=cos
  Demux1 : Demux  Outputs=2
  Display5 : Display
  Mux3 : Mux  Inputs=2
  Product{,1..3} (4 alike) : Product
  Sin : Trigonometry
  Sum : Sum
  Sum1 : Sum  Inputs=+-
  v_vsc_dq : Outport  InitialOutput=[0,0]  VectorParamsAs1DForOutWhenUnconnected=off
  wires:
  Demux1/1 -> Product/1, Product3/1
  wt/1 -> Sin/1, Cos/1
  Product/1 -> Sum/1
  Sum/1 -> Mux3/1
  Mux3/1 -> Display5/1, v_vsc_dq/1
  Sum1/1 -> Mux3/2
  v_vsc_DQ/1 -> Demux1/1
  Sin/1 -> Product1/2, Product3/2
  Product1/1 -> Sum/2
  Cos/1 -> Product/2, Product2/2
  Product2/1 -> Sum1/1
  Demux1/2 -> Product1/1, Product2/1
  Product3/1 -> Sum1/2

== system version4_dq/GFM+WT/grid>>PLL3 ==
  note: *
  note: =
  note: inv ([  cos(wt)   sin(wt)
      |    -sin(wt)    cos(wt)   ])
  note: [ d
      |    q ]
  note: [  al
      |     be  ]
  note: *
  note: =
  note: [  cos(wt)   -sin(wt)
      |    sin(wt)    cos(wt)   ]
  note: [ d
      |    q ]
  note: [  al
      |     be  ]
  v_vsc_DQref : Inport
  wt : Inport  Port=2
  Cos : Trigonometry  Operator=cos
  Demux1 : Demux  Outputs=[vect vect]
  Display5 : Display
  Mux3 : Mux  Inputs=2
  Product{,1..3} (4 alike) : Product
  Sin : Trigonometry
  Sum : Sum
  Sum1 : Sum  Inputs=+-
  vgdq : Outport  InitialOutput=[0,0]  VectorParamsAs1DForOutWhenUnconnected=off
  wires:
  Demux1/1 -> Product/1, Product3/1
  wt/1 -> Sin/1, Cos/1
  Product/1 -> Sum/1
  Sum/1 -> Mux3/1
  Mux3/1 -> Display5/1, vgdq/1
  Sum1/1 -> Mux3/2
  v_vsc_DQref/1 -> Demux1/1
  Sin/1 -> Product1/2, Product3/2
  Product1/1 -> Sum/2
  Cos/1 -> Product/2, Product2/2
  Product2/1 -> Sum1/1
  Demux1/2 -> Product1/1, Product2/1
  Product3/1 -> Sum1/2

== system version4_dq/GFM+WT/grid>>PLL4 ==
  note: *
  note: =
  note: inv ([  cos(wt)   sin(wt)
      |    -sin(wt)    cos(wt)   ])
  note: [ d
      |    q ]
  note: [  al
      |     be  ]
  note: *
  note: =
  note: [  cos(wt)   -sin(wt)
      |    sin(wt)    cos(wt)   ]
  note: [ d
      |    q ]
  note: [  al
      |     be  ]
  i_grid_DQ : Inport
  wt : Inport  Port=2
  Cos : Trigonometry  Operator=cos
  Demux1 : Demux  Outputs=[vect vect]
  Display5 : Display
  Mux3 : Mux  Inputs=2
  Product{,1..3} (4 alike) : Product
  Sin : Trigonometry
  Sum : Sum
  Sum1 : Sum  Inputs=+-
  vgdq : Outport  InitialOutput=[0,0]  VectorParamsAs1DForOutWhenUnconnected=off
  wires:
  Demux1/1 -> Product/1, Product3/1
  wt/1 -> Sin/1, Cos/1
  Product/1 -> Sum/1
  Sum/1 -> Mux3/1
  Mux3/1 -> Display5/1, vgdq/1
  Sum1/1 -> Mux3/2
  i_grid_DQ/1 -> Demux1/1
  Sin/1 -> Product1/2, Product3/2
  Product1/1 -> Sum/2
  Cos/1 -> Product/2, Product2/2
  Product2/1 -> Sum1/1
  Demux1/2 -> Product1/1, Product2/1
  Product3/1 -> Sum1/2

== system version4_dq/HVAC CABLE 10 PI SEGMENTS 1/RC sys1 ==
  note: Left shunt capacitor
  note: shunt capacitor
  Iload_DQ : Inport
  "Isource_DQ " : Inport  Port=2
  omega_ref : Inport  Port=3
  1 : Gain  Gain=Rd
  10 : Gain  Gain=inv_Csource
  2 : Gain  Gain=Rd
  8 : Gain  Gain=Csource
  9 : Gain  Gain=inv_Csource
  Demux2 : Demux  Outputs=2
  Demux3 : Demux  Outputs=2
  Display1 : Display
  Display6 : Display
  Mux1 : Mux  Inputs=2
  Mux2 : Mux  Inputs=2
  Product7 : Product
  Product8 : Product
  Sum1 : Sum  Inputs=|++
  Sum14 : Sum  Inputs=|+--
  Sum15 : Sum  Inputs=|++-
  Sum2 : Sum  Inputs=|++
  Sum3 : Sum  Inputs=|+-
  Sum4 : Sum  Inputs=|+-
  Vcd : Scope
  VcpdR_int : Integrator  InitialCondition=VD0  UpperSaturationLimit=50  LowerSaturationLimit=-1000
  VcpqR_int : Integrator  InitialCondition=VQ0  UpperSaturationLimit=50  LowerSaturationLimit=-1000
  Vcq : Scope
  VpccR_DQ : Outport  VectorParamsAs1DForOutWhenUnconnected=off
  wires:
  8/1 -> [wcs], Display1/1
  Mux1/1 -> VpccR_DQ/1
  Product8/1 -> Sum14/3
  Sum15/1 -> 9/1
  10/1 -> VcpqR_int/1
  Product7/1 -> Sum15/1
  VcpqR_int/1 -> Mux2/1, Sum2/1, Product7/2, Vcq/1
  [wcs] -> Product7/1, Product8/1
  Sum14/1 -> 10/1
  9/1 -> VcpdR_int/1
  omega_ref/1 -> 8/1
  Demux2/1 -> Sum4/1, Sum15/2
  Demux2/2 -> Sum3/1, Sum14/1
  Iload_DQ/1 -> Demux2/1
  "Isource_DQ "/1 -> Demux3/1
  Demux3/2 -> Sum3/2, Sum14/2
  Demux3/1 -> Sum4/2, Sum15/3
  VcpdR_int/1 -> Mux2/2, Product8/2, Sum1/1
  Sum1/1 -> Mux1/1
  Sum2/1 -> Mux1/2
  1/1 -> Sum2/2
  2/1 -> Sum1/2
  Mux2/1 -> Display6/1
  Sum3/1 -> 1/1
  Sum4/1 -> 2/1

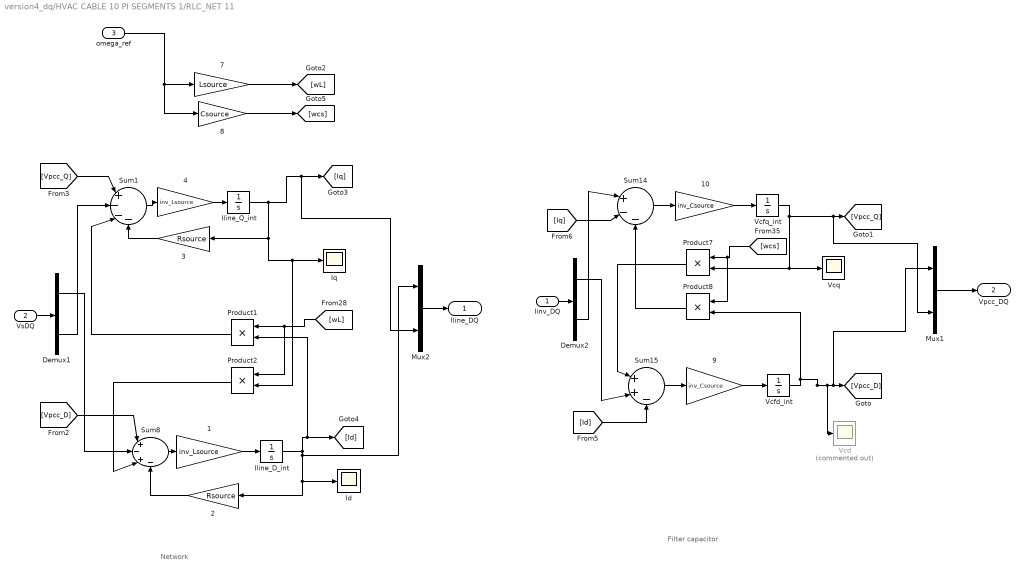
== system version4_dq/HVAC CABLE 10 PI SEGMENTS 1/RLC_NET 11 ==
  note: Network
  note: Filter capacitor
  Iinv_DQ : Inport
  "VsDQ " : Inport  Port=2
  omega_ref : Inport  Port=3
  1 : Gain  Gain=inv_Lsource
  10 : Gain  Gain=inv_Csource
  2 : Gain  Gain=Rsource
  3 : Gain  Gain=Rsource
  4 : Gain  Gain=inv_Lsource
  7 : Gain  Gain=Lsource
  8 : Gain  Gain=Csource
  9 : Gain  Gain=inv_Csource
  Demux1 : Demux  Outputs=2
  Demux2 : Demux  Outputs=2
  Id : Scope
  Iline_D_int : Integrator  UpperSaturationLimit=50  LowerSaturationLimit=-1000
  Iline_Q_int : Integrator  UpperSaturationLimit=50  LowerSaturationLimit=-1000
  Iq : Scope
  Mux1 : Mux  Inputs=2
  Mux2 : Mux  Inputs=2
  Product{1..2,7..8} (4 alike) : Product
  Sum1 : Sum  Inputs=|+---
  Sum14 : Sum  Inputs=|+--
  Sum15 : Sum  Inputs=|++-
  Sum8 : Sum  Inputs=|+-+-
  Vcd : Scope  Commented=on
  Vcfd_int : Integrator  UpperSaturationLimit=50  LowerSaturationLimit=-1000
  Vcfq_int : Integrator  UpperSaturationLimit=50  LowerSaturationLimit=-1000
  Vcq : Scope
  Iline_DQ : Outport  VectorParamsAs1DForOutWhenUnconnected=off
  Vpcc_DQ : Outport  Port=2  VectorParamsAs1DForOutWhenUnconnected=off
  wires:
  Mux2/1 -> Iline_DQ/1
  Iinv_DQ/1 -> Demux2/1
  Demux2/2 -> Sum14/1
  Demux2/1 -> Sum15/2
  [wL] -> Product2/1, Product1/1
  Product1/1 -> Sum1/3
  4/1 -> Iline_Q_int/1
  3/1 -> Sum1/4
  Product2/1 -> Sum8/3
  2/1 -> Sum8/4
  Sum8/1 -> 1/1
  Iline_Q_int/1 -> 3/1, Product2/2, Iq/1, [Iq], Mux2/2
  Iline_D_int/1 -> Mux2/1, 2/1, Id/1, Product1/2, [Id]
  1/1 -> Iline_D_int/1
  Sum1/1 -> 4/1
  [Vpcc_D] -> Sum8/1
  [Vpcc_Q] -> Sum1/1
  omega_ref/1 -> 8/1, 7/1
  7/1 -> [wL]
  9/1 -> Vcfd_int/1
  Sum14/1 -> 10/1
  [wcs] -> Product8/1, Product7/1
  [Id] -> Sum15/3
  Vcfq_int/1 -> Mux1/2, [Vpcc_Q], Product7/2, Vcq/1
  Product7/1 -> Sum15/1
  [Iq] -> Sum14/2
  10/1 -> Vcfq_int/1
  Sum15/1 -> 9/1
  Product8/1 -> Sum14/3
  8/1 -> [wcs]
  Vcfd_int/1 -> Product8/2, Mux1/1, [Vpcc_D], Vcd/1
  Mux1/1 -> Vpcc_DQ/1
  Demux1/1 -> Sum8/2
  Demux1/2 -> Sum1/2
  "VsDQ "/1 -> Demux1/1

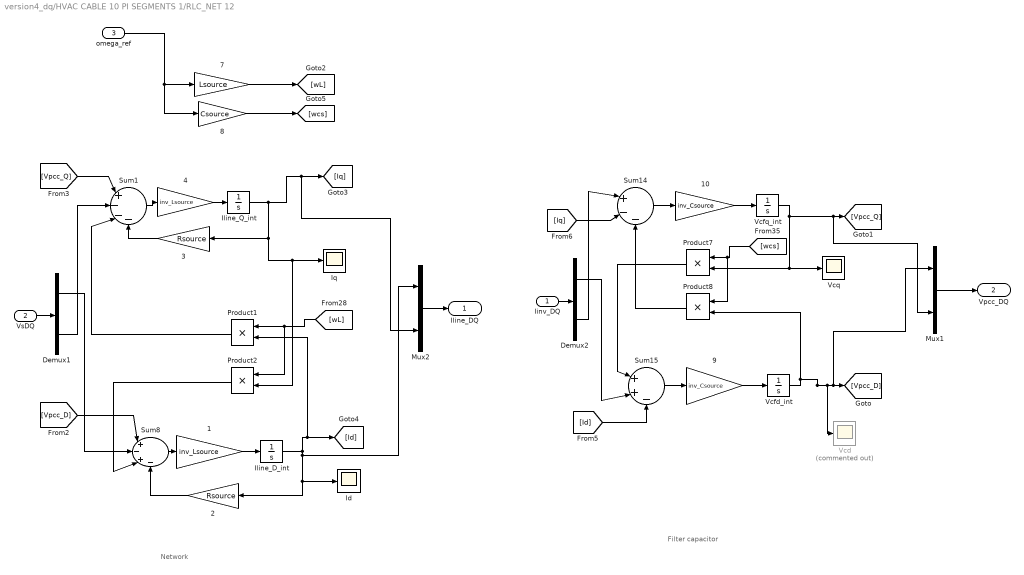
== system version4_dq/HVAC CABLE 10 PI SEGMENTS 1/RLC_NET 12 ==
  note: Filter capacitor
  note: Network
  Iinv_DQ : Inport
  "VsDQ " : Inport  Port=2
  omega_ref : Inport  Port=3
  1 : Gain  Gain=inv_Lsource
  10 : Gain  Gain=inv_Csource
  2 : Gain  Gain=Rsource
  3 : Gain  Gain=Rsource
  4 : Gain  Gain=inv_Lsource
  7 : Gain  Gain=Lsource
  8 : Gain  Gain=Csource
  9 : Gain  Gain=inv_Csource
  Demux1 : Demux  Outputs=2
  Demux2 : Demux  Outputs=2
  Id : Scope
  Iline_D_int : Integrator  UpperSaturationLimit=50  LowerSaturationLimit=-1000
  Iline_Q_int : Integrator  UpperSaturationLimit=50  LowerSaturationLimit=-1000
  Iq : Scope
  Mux1 : Mux  Inputs=2
  Mux2 : Mux  Inputs=2
  Product{1..2,7..8} (4 alike) : Product
  Sum1 : Sum  Inputs=|+---
  Sum14 : Sum  Inputs=|+--
  Sum15 : Sum  Inputs=|++-
  Sum8 : Sum  Inputs=|+-+-
  Vcd : Scope  Commented=on
  Vcfd_int : Integrator  UpperSaturationLimit=50  LowerSaturationLimit=-1000
  Vcfq_int : Integrator  UpperSaturationLimit=50  LowerSaturationLimit=-1000
  Vcq : Scope
  Iline_DQ : Outport  VectorParamsAs1DForOutWhenUnconnected=off
  Vpcc_DQ : Outport  Port=2  VectorParamsAs1DForOutWhenUnconnected=off
  wires:
  "VsDQ "/1 -> Demux1/1
  Demux1/2 -> Sum1/2
  Demux1/1 -> Sum8/2
  Mux1/1 -> Vpcc_DQ/1
  Vcfd_int/1 -> Vcd/1, [Vpcc_D], Mux1/1, Product8/2
  8/1 -> [wcs]
  Product8/1 -> Sum14/3
  Sum15/1 -> 9/1
  10/1 -> Vcfq_int/1
  [Iq] -> Sum14/2
  Product7/1 -> Sum15/1
  Vcfq_int/1 -> Vcq/1, Product7/2, [Vpcc_Q], Mux1/2
  [Id] -> Sum15/3
  [wcs] -> Product7/1, Product8/1
  Sum14/1 -> 10/1
  9/1 -> Vcfd_int/1
  7/1 -> [wL]
  omega_ref/1 -> 7/1, 8/1
  [Vpcc_Q] -> Sum1/1
  [Vpcc_D] -> Sum8/1
  Sum1/1 -> 4/1
  1/1 -> Iline_D_int/1
  Iline_D_int/1 -> [Id], Product1/2, Id/1, 2/1, Mux2/1
  Iline_Q_int/1 -> Mux2/2, [Iq], Iq/1, Product2/2, 3/1
  Sum8/1 -> 1/1
  2/1 -> Sum8/4
  Product2/1 -> Sum8/3
  3/1 -> Sum1/4
  4/1 -> Iline_Q_int/1
  Product1/1 -> Sum1/3
  [wL] -> Product1/1, Product2/1
  Demux2/1 -> Sum15/2
  Demux2/2 -> Sum14/1
  Iinv_DQ/1 -> Demux2/1
  Mux2/1 -> Iline_DQ/1

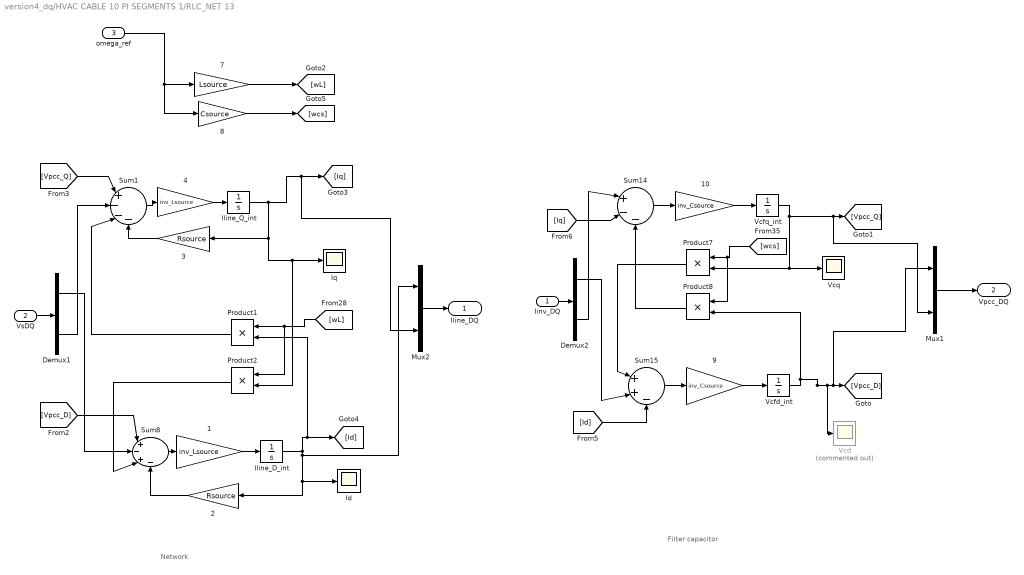
== system version4_dq/HVAC CABLE 10 PI SEGMENTS 1/RLC_NET 13 ==
  note: Filter capacitor
  note: Network
  Iinv_DQ : Inport
  "VsDQ " : Inport  Port=2
  omega_ref : Inport  Port=3
  1 : Gain  Gain=inv_Lsource
  10 : Gain  Gain=inv_Csource
  2 : Gain  Gain=Rsource
  3 : Gain  Gain=Rsource
  4 : Gain  Gain=inv_Lsource
  7 : Gain  Gain=Lsource
  8 : Gain  Gain=Csource
  9 : Gain  Gain=inv_Csource
  Demux1 : Demux  Outputs=2
  Demux2 : Demux  Outputs=2
  Id : Scope
  Iline_D_int : Integrator  UpperSaturationLimit=50  LowerSaturationLimit=-1000
  Iline_Q_int : Integrator  UpperSaturationLimit=50  LowerSaturationLimit=-1000
  Iq : Scope
  Mux1 : Mux  Inputs=2
  Mux2 : Mux  Inputs=2
  Product{1..2,7..8} (4 alike) : Product
  Sum1 : Sum  Inputs=|+---
  Sum14 : Sum  Inputs=|+--
  Sum15 : Sum  Inputs=|++-
  Sum8 : Sum  Inputs=|+-+-
  Vcd : Scope  Commented=on
  Vcfd_int : Integrator  UpperSaturationLimit=50  LowerSaturationLimit=-1000
  Vcfq_int : Integrator  UpperSaturationLimit=50  LowerSaturationLimit=-1000
  Vcq : Scope
  Iline_DQ : Outport  VectorParamsAs1DForOutWhenUnconnected=off
  Vpcc_DQ : Outport  Port=2  VectorParamsAs1DForOutWhenUnconnected=off
  wires:
  "VsDQ "/1 -> Demux1/1
  Demux1/2 -> Sum1/2
  Demux1/1 -> Sum8/2
  Mux1/1 -> Vpcc_DQ/1
  Vcfd_int/1 -> Vcd/1, [Vpcc_D], Mux1/1, Product8/2
  8/1 -> [wcs]
  Product8/1 -> Sum14/3
  Sum15/1 -> 9/1
  10/1 -> Vcfq_int/1
  [Iq] -> Sum14/2
  Product7/1 -> Sum15/1
  Vcfq_int/1 -> Vcq/1, Product7/2, [Vpcc_Q], Mux1/2
  [Id] -> Sum15/3
  [wcs] -> Product7/1, Product8/1
  Sum14/1 -> 10/1
  9/1 -> Vcfd_int/1
  7/1 -> [wL]
  omega_ref/1 -> 7/1, 8/1
  [Vpcc_Q] -> Sum1/1
  [Vpcc_D] -> Sum8/1
  Sum1/1 -> 4/1
  1/1 -> Iline_D_int/1
  Iline_D_int/1 -> [Id], Product1/2, Id/1, 2/1, Mux2/1
  Iline_Q_int/1 -> Mux2/2, [Iq], Iq/1, Product2/2, 3/1
  Sum8/1 -> 1/1
  2/1 -> Sum8/4
  Product2/1 -> Sum8/3
  3/1 -> Sum1/4
  4/1 -> Iline_Q_int/1
  Product1/1 -> Sum1/3
  [wL] -> Product1/1, Product2/1
  Demux2/1 -> Sum15/2
  Demux2/2 -> Sum14/1
  Iinv_DQ/1 -> Demux2/1
  Mux2/1 -> Iline_DQ/1

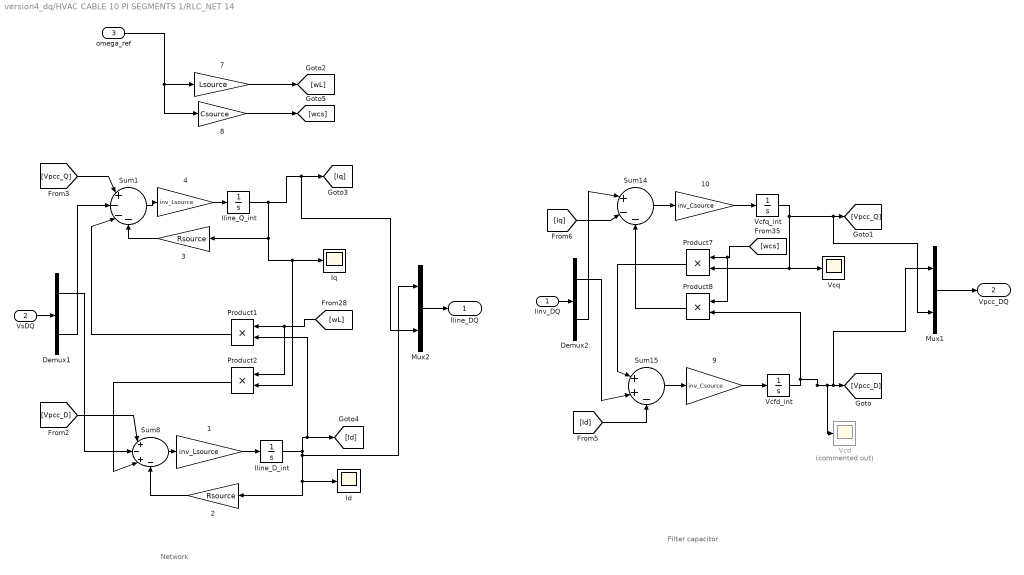
== system version4_dq/HVAC CABLE 10 PI SEGMENTS 1/RLC_NET 14 ==
  note: Network
  note: Filter capacitor
  Iinv_DQ : Inport
  "VsDQ " : Inport  Port=2
  omega_ref : Inport  Port=3
  1 : Gain  Gain=inv_Lsource
  10 : Gain  Gain=inv_Csource
  2 : Gain  Gain=Rsource
  3 : Gain  Gain=Rsource
  4 : Gain  Gain=inv_Lsource
  7 : Gain  Gain=Lsource
  8 : Gain  Gain=Csource
  9 : Gain  Gain=inv_Csource
  Demux1 : Demux  Outputs=2
  Demux2 : Demux  Outputs=2
  Id : Scope
  Iline_D_int : Integrator  UpperSaturationLimit=50  LowerSaturationLimit=-1000
  Iline_Q_int : Integrator  UpperSaturationLimit=50  LowerSaturationLimit=-1000
  Iq : Scope
  Mux1 : Mux  Inputs=2
  Mux2 : Mux  Inputs=2
  Product{1..2,7..8} (4 alike) : Product
  Sum1 : Sum  Inputs=|+---
  Sum14 : Sum  Inputs=|+--
  Sum15 : Sum  Inputs=|++-
  Sum8 : Sum  Inputs=|+-+-
  Vcd : Scope  Commented=on
  Vcfd_int : Integrator  UpperSaturationLimit=50  LowerSaturationLimit=-1000
  Vcfq_int : Integrator  UpperSaturationLimit=50  LowerSaturationLimit=-1000
  Vcq : Scope
  Iline_DQ : Outport  VectorParamsAs1DForOutWhenUnconnected=off
  Vpcc_DQ : Outport  Port=2  VectorParamsAs1DForOutWhenUnconnected=off
  wires:
  Mux2/1 -> Iline_DQ/1
  Iinv_DQ/1 -> Demux2/1
  Demux2/2 -> Sum14/1
  Demux2/1 -> Sum15/2
  [wL] -> Product2/1, Product1/1
  Product1/1 -> Sum1/3
  4/1 -> Iline_Q_int/1
  3/1 -> Sum1/4
  Product2/1 -> Sum8/3
  2/1 -> Sum8/4
  Sum8/1 -> 1/1
  Iline_Q_int/1 -> 3/1, Product2/2, Iq/1, [Iq], Mux2/2
  Iline_D_int/1 -> Mux2/1, 2/1, Id/1, Product1/2, [Id]
  1/1 -> Iline_D_int/1
  Sum1/1 -> 4/1
  [Vpcc_D] -> Sum8/1
  [Vpcc_Q] -> Sum1/1
  omega_ref/1 -> 8/1, 7/1
  7/1 -> [wL]
  9/1 -> Vcfd_int/1
  Sum14/1 -> 10/1
  [wcs] -> Product8/1, Product7/1
  [Id] -> Sum15/3
  Vcfq_int/1 -> Mux1/2, [Vpcc_Q], Product7/2, Vcq/1
  Product7/1 -> Sum15/1
  [Iq] -> Sum14/2
  10/1 -> Vcfq_int/1
  Sum15/1 -> 9/1
  Product8/1 -> Sum14/3
  8/1 -> [wcs]
  Vcfd_int/1 -> Product8/2, Mux1/1, [Vpcc_D], Vcd/1
  Mux1/1 -> Vpcc_DQ/1
  Demux1/1 -> Sum8/2
  Demux1/2 -> Sum1/2
  "VsDQ "/1 -> Demux1/1

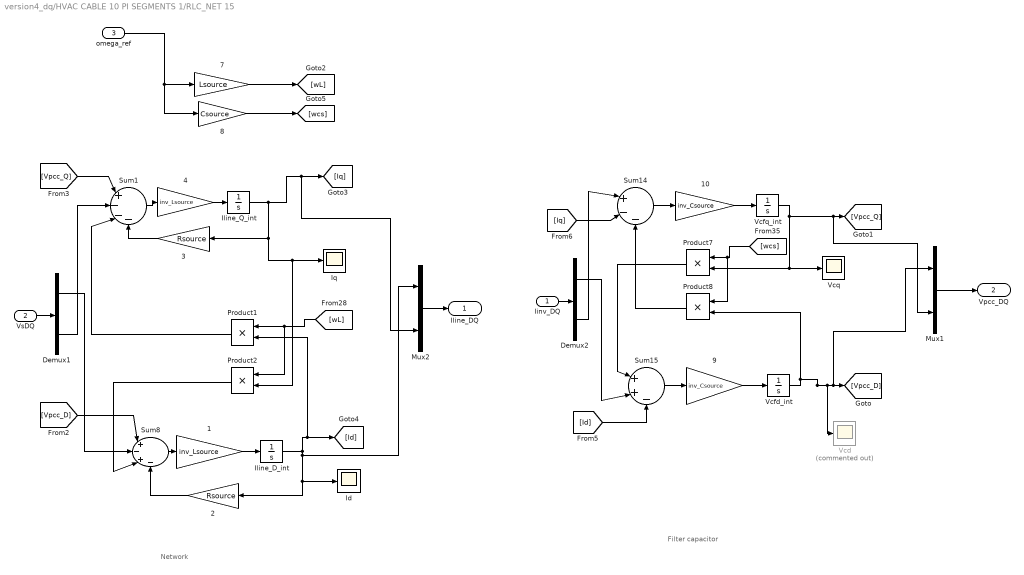
== system version4_dq/HVAC CABLE 10 PI SEGMENTS 1/RLC_NET 15 ==
  note: Filter capacitor
  note: Network
  Iinv_DQ : Inport
  "VsDQ " : Inport  Port=2
  omega_ref : Inport  Port=3
  1 : Gain  Gain=inv_Lsource
  10 : Gain  Gain=inv_Csource
  2 : Gain  Gain=Rsource
  3 : Gain  Gain=Rsource
  4 : Gain  Gain=inv_Lsource
  7 : Gain  Gain=Lsource
  8 : Gain  Gain=Csource
  9 : Gain  Gain=inv_Csource
  Demux1 : Demux  Outputs=2
  Demux2 : Demux  Outputs=2
  Id : Scope
  Iline_D_int : Integrator  UpperSaturationLimit=50  LowerSaturationLimit=-1000
  Iline_Q_int : Integrator  UpperSaturationLimit=50  LowerSaturationLimit=-1000
  Iq : Scope
  Mux1 : Mux  Inputs=2
  Mux2 : Mux  Inputs=2
  Product{1..2,7..8} (4 alike) : Product
  Sum1 : Sum  Inputs=|+---
  Sum14 : Sum  Inputs=|+--
  Sum15 : Sum  Inputs=|++-
  Sum8 : Sum  Inputs=|+-+-
  Vcd : Scope  Commented=on
  Vcfd_int : Integrator  UpperSaturationLimit=50  LowerSaturationLimit=-1000
  Vcfq_int : Integrator  UpperSaturationLimit=50  LowerSaturationLimit=-1000
  Vcq : Scope
  Iline_DQ : Outport  VectorParamsAs1DForOutWhenUnconnected=off
  Vpcc_DQ : Outport  Port=2  VectorParamsAs1DForOutWhenUnconnected=off
  wires:
  "VsDQ "/1 -> Demux1/1
  Demux1/2 -> Sum1/2
  Demux1/1 -> Sum8/2
  Mux1/1 -> Vpcc_DQ/1
  Vcfd_int/1 -> Vcd/1, [Vpcc_D], Mux1/1, Product8/2
  8/1 -> [wcs]
  Product8/1 -> Sum14/3
  Sum15/1 -> 9/1
  10/1 -> Vcfq_int/1
  [Iq] -> Sum14/2
  Product7/1 -> Sum15/1
  Vcfq_int/1 -> Vcq/1, Product7/2, [Vpcc_Q], Mux1/2
  [Id] -> Sum15/3
  [wcs] -> Product7/1, Product8/1
  Sum14/1 -> 10/1
  9/1 -> Vcfd_int/1
  7/1 -> [wL]
  omega_ref/1 -> 7/1, 8/1
  [Vpcc_Q] -> Sum1/1
  [Vpcc_D] -> Sum8/1
  Sum1/1 -> 4/1
  1/1 -> Iline_D_int/1
  Iline_D_int/1 -> [Id], Product1/2, Id/1, 2/1, Mux2/1
  Iline_Q_int/1 -> Mux2/2, [Iq], Iq/1, Product2/2, 3/1
  Sum8/1 -> 1/1
  2/1 -> Sum8/4
  Product2/1 -> Sum8/3
  3/1 -> Sum1/4
  4/1 -> Iline_Q_int/1
  Product1/1 -> Sum1/3
  [wL] -> Product1/1, Product2/1
  Demux2/1 -> Sum15/2
  Demux2/2 -> Sum14/1
  Iinv_DQ/1 -> Demux2/1
  Mux2/1 -> Iline_DQ/1

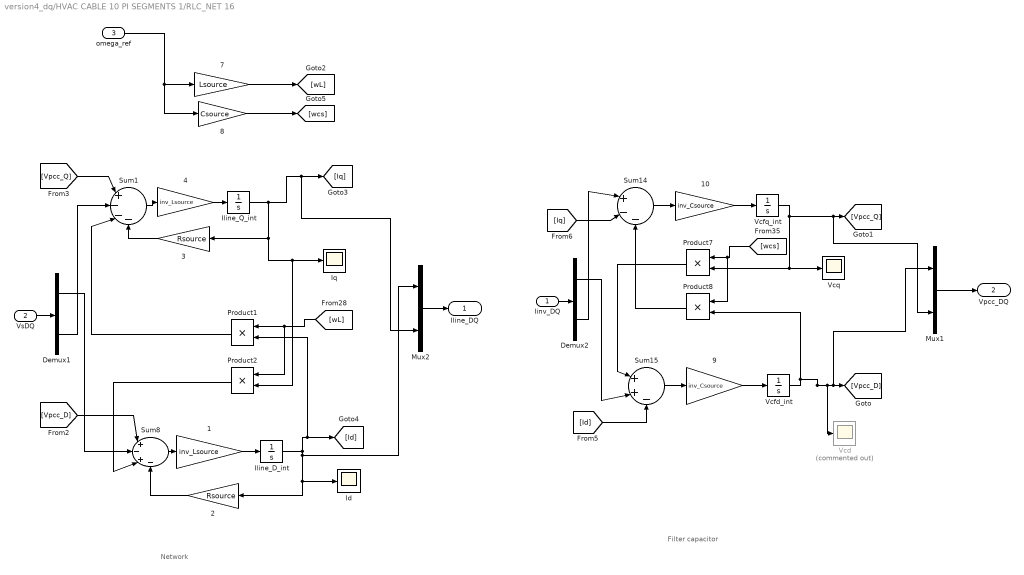
== system version4_dq/HVAC CABLE 10 PI SEGMENTS 1/RLC_NET 16 ==
  note: Filter capacitor
  note: Network
  Iinv_DQ : Inport
  "VsDQ " : Inport  Port=2
  omega_ref : Inport  Port=3
  1 : Gain  Gain=inv_Lsource
  10 : Gain  Gain=inv_Csource
  2 : Gain  Gain=Rsource
  3 : Gain  Gain=Rsource
  4 : Gain  Gain=inv_Lsource
  7 : Gain  Gain=Lsource
  8 : Gain  Gain=Csource
  9 : Gain  Gain=inv_Csource
  Demux1 : Demux  Outputs=2
  Demux2 : Demux  Outputs=2
  Id : Scope
  Iline_D_int : Integrator  UpperSaturationLimit=50  LowerSaturationLimit=-1000
  Iline_Q_int : Integrator  UpperSaturationLimit=50  LowerSaturationLimit=-1000
  Iq : Scope
  Mux1 : Mux  Inputs=2
  Mux2 : Mux  Inputs=2
  Product{1..2,7..8} (4 alike) : Product
  Sum1 : Sum  Inputs=|+---
  Sum14 : Sum  Inputs=|+--
  Sum15 : Sum  Inputs=|++-
  Sum8 : Sum  Inputs=|+-+-
  Vcd : Scope  Commented=on
  Vcfd_int : Integrator  UpperSaturationLimit=50  LowerSaturationLimit=-1000
  Vcfq_int : Integrator  UpperSaturationLimit=50  LowerSaturationLimit=-1000
  Vcq : Scope
  Iline_DQ : Outport  VectorParamsAs1DForOutWhenUnconnected=off
  Vpcc_DQ : Outport  Port=2  VectorParamsAs1DForOutWhenUnconnected=off
  wires:
  "VsDQ "/1 -> Demux1/1
  Demux1/2 -> Sum1/2
  Demux1/1 -> Sum8/2
  Mux1/1 -> Vpcc_DQ/1
  Vcfd_int/1 -> Vcd/1, [Vpcc_D], Mux1/1, Product8/2
  8/1 -> [wcs]
  Product8/1 -> Sum14/3
  Sum15/1 -> 9/1
  10/1 -> Vcfq_int/1
  [Iq] -> Sum14/2
  Product7/1 -> Sum15/1
  Vcfq_int/1 -> Vcq/1, Product7/2, [Vpcc_Q], Mux1/2
  [Id] -> Sum15/3
  [wcs] -> Product7/1, Product8/1
  Sum14/1 -> 10/1
  9/1 -> Vcfd_int/1
  7/1 -> [wL]
  omega_ref/1 -> 7/1, 8/1
  [Vpcc_Q] -> Sum1/1
  [Vpcc_D] -> Sum8/1
  Sum1/1 -> 4/1
  1/1 -> Iline_D_int/1
  Iline_D_int/1 -> [Id], Product1/2, Id/1, 2/1, Mux2/1
  Iline_Q_int/1 -> Mux2/2, [Iq], Iq/1, Product2/2, 3/1
  Sum8/1 -> 1/1
  2/1 -> Sum8/4
  Product2/1 -> Sum8/3
  3/1 -> Sum1/4
  4/1 -> Iline_Q_int/1
  Product1/1 -> Sum1/3
  [wL] -> Product1/1, Product2/1
  Demux2/1 -> Sum15/2
  Demux2/2 -> Sum14/1
  Iinv_DQ/1 -> Demux2/1
  Mux2/1 -> Iline_DQ/1
